simulink model "week2problem3"  (R2020b)
settings: Solver=VariableStepAuto  StartTime=0.0  StopTime=120  RelTol=1e-3
model workspace (MAT data in the model file):
  b = 50
  m = 1000
  u = 500
settings Model: DataDictionary=parameter3.sldd  Creator=Puru Gawande  LastModifiedBy=Puru Gawande

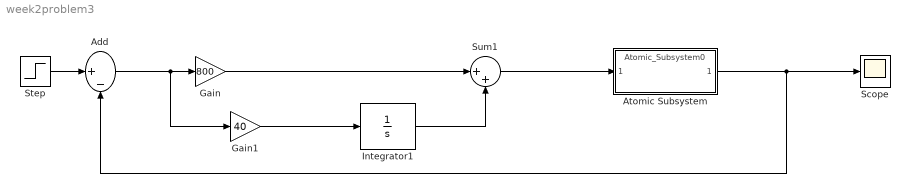
== system week2problem3 ==
  Add : Sum  Inputs=|+-
  Atomic Subsystem : ModelReference  ModelNameDialog=Atomic_Subsystem0  SimulationMode=Normal  ModelReferenceVersion=1.11
  Gain : Gain  Gain=800
  Gain1 : Gain  Gain=40
  Integrator1 : Integrator
  Scope : Scope
  Step : Step  Time=0  After=u  SampleTime=0
  Sum1 : Sum  Inputs=|++
  wires:
  Integrator1/1 -> Sum1/2
  Gain/1 -> Sum1/1
  Gain1/1 -> Integrator1/1
  Sum1/1 -> Atomic Subsystem/1
  Atomic Subsystem/1 -> Add/2, Scope/1
  Step/1 -> Add/1
  Add/1 -> Gain1/1, Gain/1
